simulink model "FIR_LMS"  (R2022a)
settings: Solver=FixedStepDiscrete  StartTime=0.0  StopTime=100e-6  RelTol=1e-3
undefined symbols (not defined in the file or in its folder): xc7k160tfbg676
libraries: hdlBasic x67, vmcUtilities x1
settings Model: Creator=gaherere  LastModifiedBy=Daniel
settings DebuggingCC: UnconnectedInputMsg=warning  UnconnectedOutputMsg=warning  UnconnectedLineMsg=warning
settings RTWCC: DLArmComputeVersion=19.05

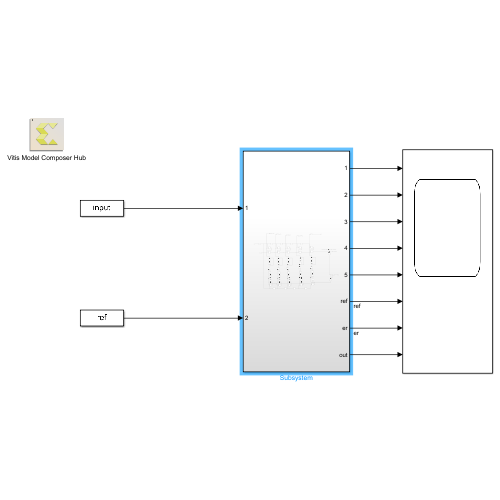
[thumbnail: Simulink's stored preview of the top-level diagram]
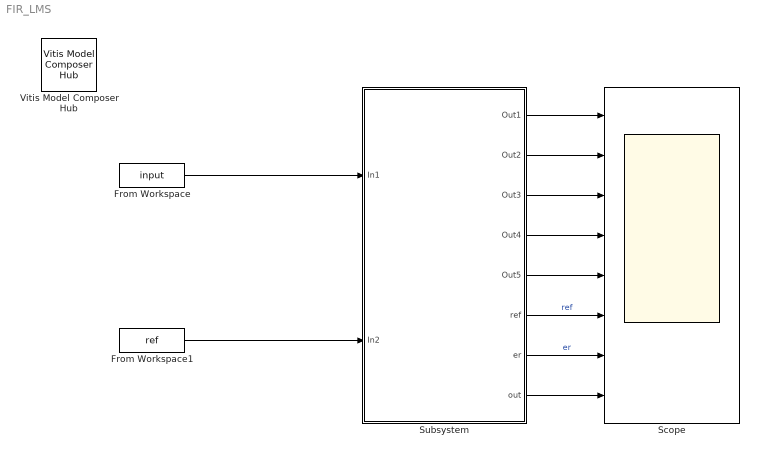
== system FIR_LMS ==
  From Workspace : FromWorkspace  VariableName=input  ZeroCross=off
  From Workspace1 : FromWorkspace  VariableName=ref  ZeroCross=off
  Scope : Scope  NumInputPorts=8
  Subsystem : Subsystem
  Vitis Model Composer Hub : vmcUtilities/Vitis Model Composer Hub  Tag=genX  CodeGeneration=off  TargetDirectory=./code  ExportType=AI Engines  IpVendor=xilinx.com  IpLibrary=hls  IpVersion=1.0  IpHWLanguage=Verilog  AieCompilerOptions={}  CreateTestbench=off  TestbenchStackSize=10  RunAieSim=off  AieSimTimeout=50000  RunAieSimProfiling=off  LaunchVitisAnalyzer=off  PlotOutput=off  RunX86Sim=off  X86SimTimeout=10  GenHwImage=off  PlatformType=Not Specified  HwSystemType=Baremetal  HwValidationTarget=hw  ProjDevice=xc7k160tfbg676-3  ProjDevicePart=xc7k160tfbg676-3  SamplePeriod=-1  ClockFrequency=200  DataPathParallelism=1  xilinxfamily=kintex7  part=xc7k160t  speed=-3  package=fbg676  directory=./netlist  testbench=off  incr_netlist=off  synthesis_tool=Vivado  clock_wrapper=Clock Enables  dbl_ovrd=According to Block Masks  dcm_input_clock_period=10  sysclk_period=50  simulink_period=50e-9  eval_field=0  IPInfoJsonString="{\"HDLSubsystem\":{\"SubsystemName\":\"Subsystem\",\"IPName\":\"Subsystem\",\"IPLibrary\":\"VMC\",\"IPVendor\":\"User Company\",\"IPVersion\":\"1.0\"}}"
  wires:
  Subsystem/1(Out1) -> Scope/1
  Subsystem/2(Out2) -> Scope/2
  Subsystem/3(Out3) -> Scope/3
  Subsystem/4(Out4) -> Scope/4
  Subsystem/5(Out5) -> Scope/5
  From Workspace/1 -> Subsystem/1(In1)
  From Workspace1/1 -> Subsystem/2(In2)
  Subsystem/7(er) -> Scope/7  "er"
  Subsystem/6(ref) -> Scope/6  "ref"
  Subsystem/8(out) -> Scope/8

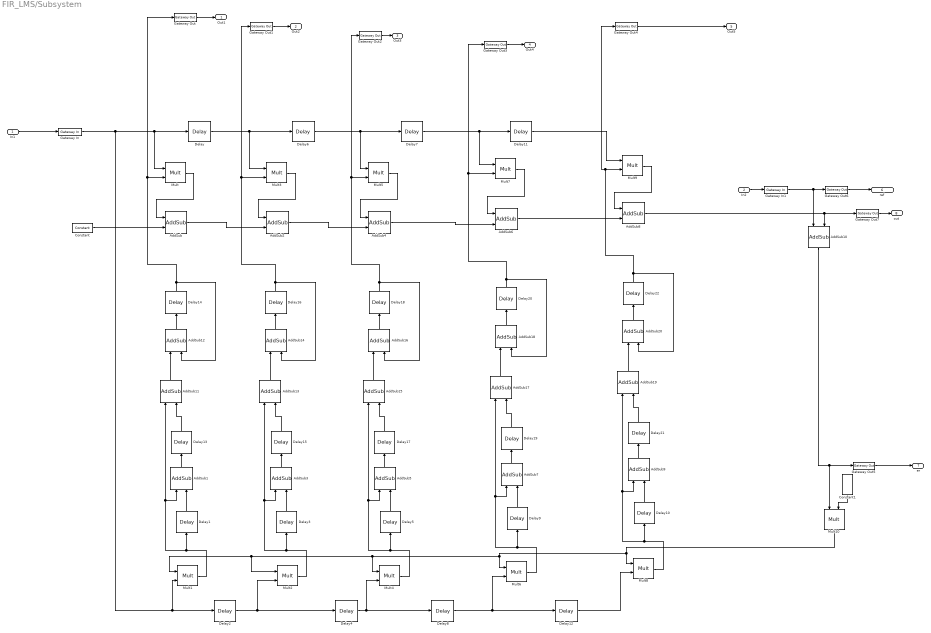
== system FIR_LMS/Subsystem ==
  In1 : Inport
  In2 : Inport  Port=2
  AddSub{,1..9,11..20} (20 alike) : hdlBasic/AddSub  mode=Addition  use_carryin=off  use_carryout=off  en=off  latency=0  precision=User Defined  arith_type="Signed  (2's comp)"  n_bits=16  bin_pt=14  quantization="Round  (unbiased: +/- Inf)"  overflow=Saturate  use_behavioral_HDL=off  hw_selection=Fabric  pipelined=off  XmcBlockStatus=1  maskContainerNames=tabcontainer1  block_type=addsub  block_config=sysgen:Addsub_config
  AddSub10 : hdlBasic/AddSub  mode=Subtraction  use_carryin=off  use_carryout=off  en=off  latency=0  precision=User Defined  arith_type="Signed  (2's comp)"  n_bits=16  bin_pt=14  quantization="Round  (unbiased: +/- Inf)"  overflow=Saturate  use_behavioral_HDL=off  hw_selection=Fabric  pipelined=off  XmcBlockStatus=1  maskContainerNames=tabcontainer1  block_type=addsub  block_config=sysgen:Addsub_config
  Constant : hdlBasic/Constant  const=0  gui_display_data_type=Fixed-point  arith_type=Signed (2's comp)  n_bits=16  bin_pt=14  preci_type=Single  exp_width=8  frac_width=24  explicit_period=off  period=1  XmcBlockStatus=1  maskContainerNames=tabcontainer1  block_type=constant  block_config=sysgen:Constant_config
  Constant1 : hdlBasic/Constant  const=0.25  gui_display_data_type=Fixed-point  arith_type=Signed (2's comp)  n_bits=16  bin_pt=14  preci_type=Single  exp_width=8  frac_width=24  explicit_period=off  period=1  XmcBlockStatus=1  maskContainerNames=tabcontainer1  block_type=constant  block_config=sysgen:Constant_config
  Delay{,1..22} (23 alike) : hdlBasic/Delay  rst=off  en=off  latency=1  reg_retiming=off  XmcBlockStatus=1  maskContainerNames=group1  block_type=delay  block_config=sysgen:Delay_config
  Gateway In : hdlBasic/Gateway In  gui_display_data_type=Fixed-point  arith_type=Signed (2's comp)  n_bits=16  bin_pt=14  preci_type=Single  exp_width=8  frac_width=24  rows=1  columns=1  quantization="Round  (unbiased: +/- Inf)"  overflow=Saturate  period=1/20e6  UseAsADC=off  ADCChannel='1'  interface=None  automatic_assignment=on  address_offset=hex2dec('00')  intf_name=''  intf_description=''  default_value=0  timing_constraint=None  locs_specified=off  LOCs={}  io_standard={}  inherit_from_input=off  hdl_port=on  XmcBlockStatus=1  maskContainerNames=group4  block_type=gatewayin  block_config=sysgen:gateway_in_config  block_width_w=590  block_height_w=620  block_width=640  block_height=850
  Gateway In1 : hdlBasic/Gateway In  gui_display_data_type=Fixed-point  arith_type=Signed (2's comp)  n_bits=16  bin_pt=14  preci_type=Single  exp_width=8  frac_width=24  rows=1  columns=1  quantization="Round  (unbiased: +/- Inf)"  overflow=Saturate  period=1/20e6  UseAsADC=off  ADCChannel='1'  interface=None  automatic_assignment=on  address_offset=hex2dec('00')  intf_name=''  intf_description=''  default_value=0  timing_constraint=None  locs_specified=off  LOCs={}  io_standard={}  inherit_from_input=off  hdl_port=on  XmcBlockStatus=1  maskContainerNames=group4  block_type=gatewayin  block_config=sysgen:gateway_in_config  block_width_w=590  block_height_w=620  block_width=640  block_height=850
  Gateway Out{,1..7} (8 alike) : hdlBasic/Gateway Out  inherit_from_input=off  hdl_port=on  rows=1  columns=1  UseAsDAC=off  DACChannel='1'  interface=None  automatic_assignment=on  address_offset=hex2dec('00')  intf_name=''  intf_description=''  timing_constraint=None  locs_specified=off  LOCs={}  io_standard={}  XmcBlockStatus=1  maskContainerNames=group4  block_type=gatewayout  block_config=sysgen:gateway_out_config  block_width_w=590  block_height_w=620  block_width=620  block_height=750
  Mult{,1..10} (11 alike) : hdlBasic/Mult  precision=User Defined  arith_type="Signed  (2's comp)"  n_bits=16  bin_pt=14  quantization="Round  (unbiased: +/- Inf)"  overflow=Saturate  en=off  latency=0  use_behavioral_HDL=off  opt=Speed  use_embedded=on  optimum_pipeline=off  pipeline=on  use_rpm=on  placement_style=Triangular  XmcBlockStatus=1  maskContainerNames=group1  block_type=mult  block_config=sysgen:Mult_config  block_width=598  block_height=876
  Out1 : Outport
  Out2 : Outport  Port=2
  Out3 : Outport  Port=3
  Out4 : Outport  Port=4
  Out5 : Outport  Port=5
  ref : Outport  Port=6
  er : Outport  Port=7
  out : Outport  Port=8
  wires:
  Delay/1 -> Delay6/1, Mult3/1
  Constant/1 -> AddSub/2
  Mult10/1 -> Mult8/1, Mult6/1, Mult4/1, Mult1/1, Mult2/1
  Constant1/1 -> Mult10/2
  Mult3/1 -> AddSub2/1
  Delay8/1 -> Delay12/1, Mult6/2
  AddSub2/1 -> AddSub4/2
  Delay12/1 -> Mult8/2
  AddSub4/1 -> AddSub6/2
  AddSub10/1 -> Mult10/1, Gateway Out5/1
  Mult5/1 -> AddSub4/1
  Delay4/1 -> Delay8/1, Mult4/2
  Delay2/1 -> Mult2/2, Delay4/1
  In2/1 -> Gateway In1/1
  Gateway In/1 -> Mult1/2, Delay2/1, Delay/1, Mult/1
  Delay6/1 -> Delay7/1, Mult5/1
  Delay11/1 -> Mult9/1
  AddSub6/1 -> AddSub8/2
  Mult/1 -> AddSub/1
  Delay7/1 -> Delay11/1, Mult7/1
  Mult9/1 -> AddSub8/1
  AddSub8/1 -> Gateway Out7/1, AddSub10/2
  Mult7/1 -> AddSub6/1
  Gateway In1/1 -> Gateway Out6/1, AddSub10/1
  AddSub/1 -> AddSub2/2
  In1/1 -> Gateway In/1
  Gateway Out/1 -> Out1/1
  Gateway Out1/1 -> Out2/1
  Gateway Out2/1 -> Out3/1
  Gateway Out3/1 -> Out4/1
  Gateway Out4/1 -> Out5/1
  Gateway Out5/1 -> er/1
  Gateway Out6/1 -> ref/1
  Gateway Out7/1 -> out/1
  Mult1/1 -> AddSub11/1, AddSub1/1, Delay1/1
  Delay1/1 -> AddSub1/2
  AddSub1/1 -> Delay13/1
  Delay13/1 -> AddSub11/2
  AddSub11/1 -> AddSub12/1
  AddSub12/1 -> Delay14/1
  Delay14/1 -> Gateway Out/1, Mult/2, AddSub12/2
  Mult2/1 -> AddSub13/1, AddSub3/1, Delay3/1
  Delay3/1 -> AddSub3/2
  Delay15/1 -> AddSub13/2
  AddSub13/1 -> AddSub14/1
  AddSub3/1 -> Delay15/1
  Delay16/1 -> Mult3/2, Gateway Out1/1, AddSub14/2
  AddSub14/1 -> Delay16/1
  Mult4/1 -> AddSub15/1, AddSub5/1, Delay5/1
  Delay5/1 -> AddSub5/2
  Delay17/1 -> AddSub15/2
  AddSub15/1 -> AddSub16/1
  AddSub5/1 -> Delay17/1
  Delay18/1 -> Gateway Out2/1, Mult5/2, AddSub16/2
  AddSub16/1 -> Delay18/1
  Mult6/1 -> AddSub17/1, AddSub7/1, Delay9/1
  Delay9/1 -> AddSub7/2
  Delay19/1 -> AddSub17/2
  AddSub17/1 -> AddSub18/1
  AddSub7/1 -> Delay19/1
  Delay20/1 -> Gateway Out3/1, Mult7/2, AddSub18/2
  AddSub18/1 -> Delay20/1
  Mult8/1 -> AddSub19/1, AddSub9/1, Delay10/1
  Delay10/1 -> AddSub9/2
  Delay21/1 -> AddSub19/2
  AddSub19/1 -> AddSub20/1
  AddSub9/1 -> Delay21/1
  Delay22/1 -> Gateway Out4/1, Mult9/2, AddSub20/2
  AddSub20/1 -> Delay22/1
